simulink model "Perfect_power_estimator"  (R2015a)
settings: Solver=ode3  StartTime=0.0  StopTime=3  FixedStep=Ts/10  RelTol=1e-3
values from neighbouring files (symbols this model uses):
  w = 2*pi*f    (= 314.159265359)    [VOC_param.m]    (also in controller_parameters.m; current_controller_param.m; power_control_param.m)
settings Model: Creator=rblan  LastModifiedBy=rblan

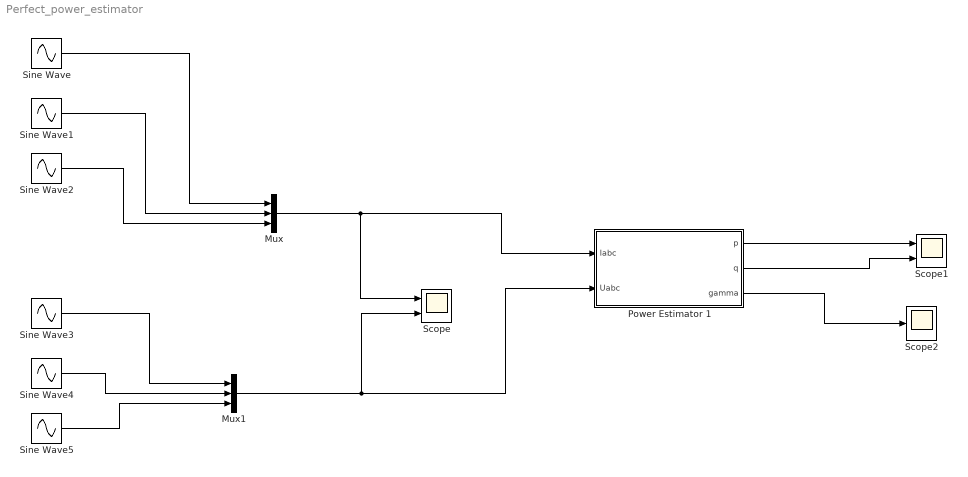
== system Perfect_power_estimator ==
  Mux : Mux  Inputs=3
  Mux1 : Mux  Inputs=3
  Power Estimator 1 : Subsystem
  Scope : Scope  NumInputPorts=2
      settings: YMin=-5~-5  YMax=5~5
  Scope1 : Scope  NumInputPorts=2
      settings: YMin=0~-8e-17  YMax=2~8e-17
  Scope2 : Scope
      settings: SaveName=ScopeData4
  Sine Wave : Sin  Frequency=w  SampleTime=0
  Sine Wave1 : Sin  Frequency=w  Phase=-2*pi/3  SampleTime=0
  Sine Wave2 : Sin  Frequency=w  Phase=-4*pi/3  SampleTime=0
  Sine Wave3 : Sin  Amplitude=0.5  Frequency=w  Phase=pi/8  SampleTime=0
  Sine Wave4 : Sin  Amplitude=0.5  Frequency=w  Phase=-2*pi/3+pi/8  SampleTime=0
  Sine Wave5 : Sin  Amplitude=0.5  Frequency=w  Phase=-4*pi/3+pi/8  SampleTime=0
  wires:
  Mux/1 -> Scope/1, Power Estimator 1/1("Iabc ")
  Sine Wave/1 -> Mux/1
  Sine Wave1/1 -> Mux/2
  Sine Wave2/1 -> Mux/3
  Mux1/1 -> Scope/2, Power Estimator 1/2("Uabc ")
  Sine Wave3/1 -> Mux1/1
  Sine Wave4/1 -> Mux1/2
  Sine Wave5/1 -> Mux1/3
  Power Estimator 1/1(p) -> Scope1/1
  Power Estimator 1/2(q) -> Scope1/2
  Power Estimator 1/3(gamma) -> Scope2/1

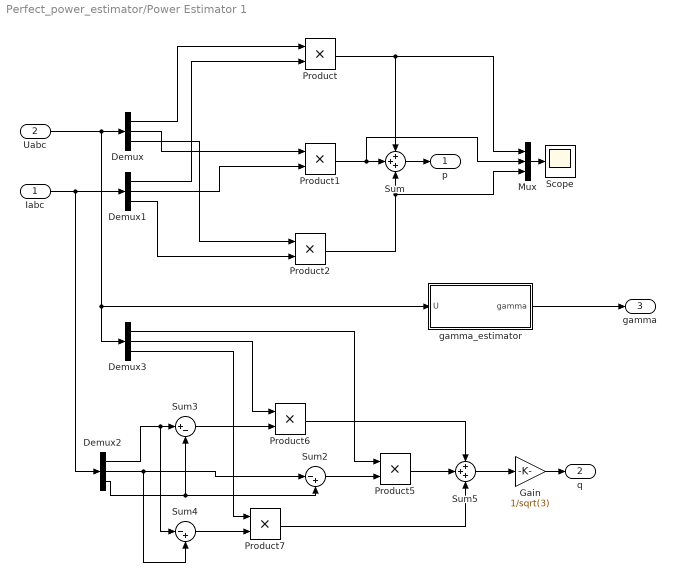
== system Perfect_power_estimator/Power Estimator 1 ==
  "Iabc " : Inport
  "Uabc " : Inport  Port=2
  Demux{,1..3} (4 alike) : Demux  Outputs=3
  Gain : Gain  Gain=1/sqrt(3)
  Mux : Mux  Inputs=3
  Product{,1..2,5..7} (6 alike) : Product
  Scope : Scope
      settings: SaveName=ScopeData5
  Sum : Sum  Inputs=+++
  Sum2 : Sum  Inputs=|-+
  Sum3 : Sum  Inputs=|+-
  Sum4 : Sum  Inputs=|-+
  Sum5 : Sum  Inputs=+++
  "gamma_estimator " : Subsystem
  p : Outport
  q : Outport  Port=2
  gamma : Outport  Port=3
  wires:
  "Uabc "/1 -> Demux3/1, "gamma_estimator "/1(U), Demux/1
  "Iabc "/1 -> Demux2/1, Demux1/1
  Demux/1 -> Product/1
  Demux1/1 -> Product/2
  Demux/2 -> Product1/1
  Demux1/2 -> Product1/2
  Demux/3 -> Product2/1
  Demux1/3 -> Product2/2
  Product1/1 -> Mux/2, Sum/2
  Product2/1 -> Mux/3, Sum/3
  Sum/1 -> p/1
  Demux2/3 -> Sum3/2, Sum2/2
  Demux2/2 -> Sum4/2, Sum2/1
  Sum2/1 -> Product5/2
  Demux3/1 -> Product5/1
  Demux2/1 -> Sum4/1, Sum3/1
  Sum3/1 -> Product6/2
  Demux3/2 -> Product6/1
  Sum4/1 -> Product7/2
  Demux3/3 -> Product7/1
  Product5/1 -> Sum5/2
  Product6/1 -> Sum5/1
  Product7/1 -> Sum5/3
  Sum5/1 -> Gain/1
  Gain/1 -> q/1
  "gamma_estimator "/1(gamma) -> gamma/1
  Mux/1 -> Scope/1
  Product/1 -> Sum/1, Mux/1

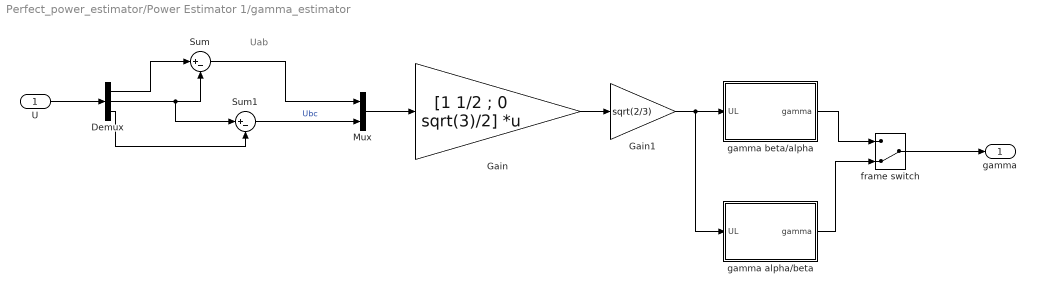
== system Perfect_power_estimator/Power Estimator 1/gamma_estimator  ==
  note: Uab
  U : Inport
  Demux : Demux  Outputs=3
  Gain : Gain  Gain=[1 1/2 ; 0 sqrt(3)/2]  Multiplication=Matrix(K*u)
  Gain1 : Gain  Gain=sqrt(2/3)
  Mux : Mux  Inputs=2
  Sum : Sum  Inputs=|+-
  Sum1 : Sum  Inputs=|+-
  frame switch : ManualSwitch  CurrentSetting=0
  gamma alpha/beta : Subsystem
  gamma beta/alpha : Subsystem
  gamma : Outport
  wires:
  Gain/1 -> Gain1/1
  Mux/1 -> Gain/1
  Sum/1 -> Mux/1
  Sum1/1 -> Mux/2  "Ubc"
  Gain1/1 -> gamma alpha/beta/1(UL), gamma beta/alpha/1(UL)
  U/1 -> Demux/1
  Demux/1 -> Sum/1
  Demux/2 -> Sum1/1, Sum/2
  Demux/3 -> Sum1/2
  gamma alpha/beta/1(gamma) -> frame switch/2
  frame switch/1 -> gamma/1
  gamma beta/alpha/1(gamma) -> frame switch/1

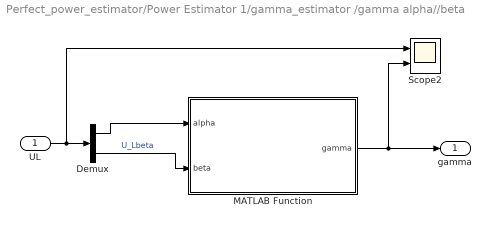
== system Perfect_power_estimator/Power Estimator 1/gamma_estimator /gamma alpha//beta ==
  UL : Inport
  Demux : Demux  Outputs=2
  MATLAB Function : MATLAB Function  TreatAsAtomicUnit=on
  Scope2 : Scope  NumInputPorts=2
      settings: TimeRange=10  YMin=-1.75~-500  YMax=1.75~300  SaveName=ScopeData15
  gamma : Outport
  wires:
  UL/1 -> Scope2/1, Demux/1
  Demux/1 -> MATLAB Function/1(alpha)
  Demux/2 -> MATLAB Function/2(beta)  "U_Lbeta"
  MATLAB Function/1(gamma) -> gamma/1, Scope2/2

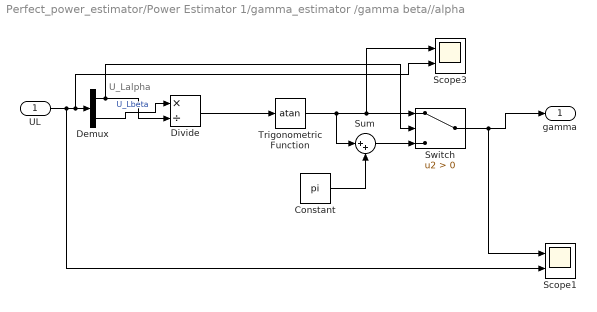
== system Perfect_power_estimator/Power Estimator 1/gamma_estimator /gamma beta//alpha ==
  note: U_Lalpha
  UL : Inport
  Constant : Constant  Value=pi
  Demux : Demux  Outputs=2
  Divide : Product  Inputs=*/
  Scope1 : Scope  NumInputPorts=2
      settings: ShowLegends=on  YMin=-2~-1.25  YMax=5~2  SaveName=ScopeData3
  Scope3 : Scope  NumInputPorts=2
      settings: YMin=-1.75~-500  YMax=1.75~300  SaveName=ScopeData2
  Sum : Sum  Inputs=|++
  Switch : Switch  Criteria=u2 > Threshold
  Trigonometric Function : Trigonometry  Operator=atan
  gamma : Outport
  wires:
  UL/1 -> Scope1/2, Scope3/2, Demux/1
  Demux/1 -> Divide/2, Switch/2
  Demux/2 -> Divide/1  "U_Lbeta"
  Constant/1 -> Sum/2
  Divide/1 -> Trigonometric Function/1
  Trigonometric Function/1 -> Sum/1, Scope3/1, Switch/1
  Sum/1 -> Switch/3
  Switch/1 -> Scope1/1, gamma/1

== matlab function Perfect_power_estimator/Power Estimator 1/gamma_estimator /gamma alpha//beta/MATLAB Function ==
  data: alpha input; gamma output; beta input
function gamma = gamma_estimator(alpha,beta)
%#codegen

gamma = 0 ; 
gamma = atan(beta/alpha) ; 

if (alpha<0 )
    gamma = gamma +pi ; 
end 

if (beta<0 && alpha> 0 ) 
    gamma = gamma +2*pi ; 
end
